simulink model "PlanarArmAug"  (R2025b)
settings: Solver=VariableStepAuto  StartTime=0.0  StopTime=10.0  RelTol=1e-3
undefined symbols (not defined in the file): InvDynAug, Jr, sig4, ureal, uss
libraries: RCTblocks x149
(part 1 of 2)
settings Model: Creator=d.alazard  LastModifiedBy=andre
settings SolverCC: AlgebraicLoopSolver=TrustRegion
settings DebuggingCC: AlgebraicLoopMsg=none  UnconnectedInputMsg=warning  UnconnectedOutputMsg=warning  UnconnectedLineMsg=warning
settings ModelReferenceCC: EnableRefExpFcnMdlSchedulingChecks=on
settings RTWCC: GPUComputeCapability=3.5  DLArmComputeVersion=19.05

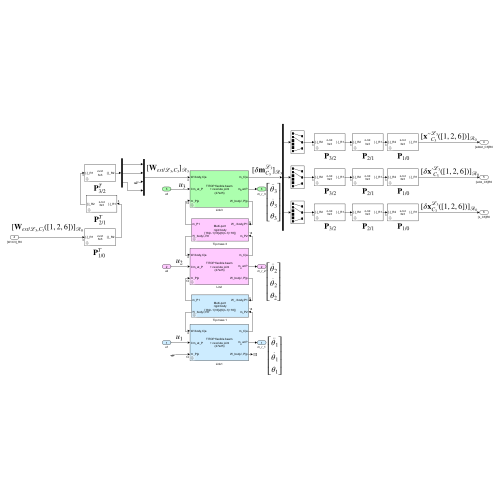
[thumbnail: Simulink's stored preview of the top-level diagram]
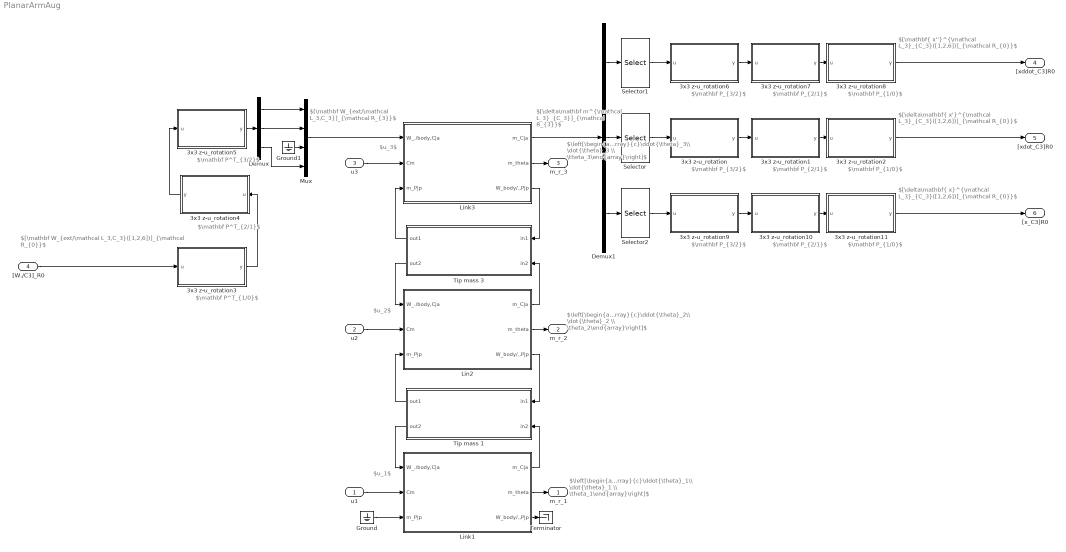
== system PlanarArmAug ==
  note: $[\delta\mathbf m^{\mathcal L_3}_{C_3}]_{\mathcal R_{3}}$
  note: $[\delta\mathbf{ x'}^{\mathcal L_3}_{C_3}([1,2,6])]_{\mathcal R_{0}}$
  note: $[\mathbf W_{ext/\mathcal L_3,C_3}]_{\mathcal R_{3}}$
  note: $[\mathbf W_{ext/\mathcal L_3,C_3}([1,2,6])]_{\mathcal R_{0}}$
  note: $u_3$
  note: $u_2$
  note: $u_1$
  note: $\left[\begin{array}{c}\ddot{\theta}_1\\ \dot{\theta}_1 \\ \theta_1\end{array}\right]$
  note: $\mathbf P_{3/2}$
  note: $\mathbf P^T_{2/1}$
  note: $\mathbf P_{1/0}$
  note: $\mathbf P^T_{1/0}$
  note: $\mathbf P_{2/1}$
  note: $\mathbf P^T_{3/2}$
  note: $\left[\begin{array}{c}\ddot{\theta}_2\\ \dot{\theta}_2 \\ \theta_2\end{array}\right]$
  note: $\left[\begin{array}{c}\ddot{\theta}_3\\ \dot{\theta}_3 \\ \theta_3\end{array}\right]$
  note: $[\mathbf{ x''}^{\mathcal L_3}_{C_3}([1,2,6])]_{\mathcal R_{0}}$
  note: $\mathbf P_{3/2}$
  note: $\mathbf P_{1/0}$
  note: $\mathbf P_{2/1}$
  note: $[\delta\mathbf{ x}^{\mathcal L_3}_{C_3}([1,2,6])]_{\mathcal R_{0}}$
  note: $\mathbf P_{3/2}$
  note: $\mathbf P_{1/0}$
  note: $\mathbf P_{2/1}$
  u1 : Inport
  u2 : Inport  Port=2
  u3 : Inport  Port=3
  "[W./C3]_R0" : Inport  Port=4
  3x3 z-u_rotation : Subsystem  mask(3x3 rotation matrix (around 3-rd axis)){theta=ureal('theta3',0,'Range',[-pi pi]), transp=off}
      mask prompts: theta "Angle (rad)"; transp "DCM transposed"
      mask help:
      | Implement the 3x3 direction cosine matrix or its transposed
      | (DCM=[cos(x)   -sin(x) 0;sin(x)  cos(x) 0;0 0 1])
      | associated to the rotation of a given angle x around the 3-rd axis.
      |
      | Angle  (rad) can be an uncertain parameter declared with "ureal" with mode 'Range'
      | Ex: ureal('NAME',0,'Range',[-pi pi])
      | Then, ULINEARIZE will provide a model involving the block named "tan_NAME_div4".
      mask init:
      | zUrotation3x3
      mask Help: web('Doc3zurotation.html','-browser')
      mask Display:
      | disp('z-rot\n3x3')
      | if transp
      |     port_label('input', 1, '[.]_R1')
      |     port_label('output', 1, '[.]_R2')
      | else
      |     port_label('input', 1, '[.]_R2')
      |     port_label('output', 1, '[.]_R1')
      | end
  3x3 z-u_rotation1 : Subsystem  mask(3x3 rotation matrix (around 3-rd axis)){theta=ureal('theta2',0,'Range',[-pi pi]), transp=off}
      mask prompts: theta "Angle (rad)"; transp "DCM transposed"
      mask help:
      | Implement the 3x3 direction cosine matrix or its transposed
      | (DCM=[cos(x)   -sin(x) 0;sin(x)  cos(x) 0;0 0 1])
      | associated to the rotation of a given angle x around the 3-rd axis.
      |
      | Angle  (rad) can be an uncertain parameter declared with "ureal" with mode 'Range'
      | Ex: ureal('NAME',0,'Range',[-pi pi])
      | Then, ULINEARIZE will provide a model involving the block named "tan_NAME_div4".
      mask init:
      | zUrotation3x3
      mask Help: web('Doc3zurotation.html','-browser')
      mask Display:
      | disp('z-rot\n3x3')
      | if transp
      |     port_label('input', 1, '[.]_R1')
      |     port_label('output', 1, '[.]_R2')
      | else
      |     port_label('input', 1, '[.]_R2')
      |     port_label('output', 1, '[.]_R1')
      | end
  3x3 z-u_rotation10 : Subsystem  mask(3x3 rotation matrix (around 3-rd axis)){theta=ureal('theta2',0,'Range',[-pi pi]), transp=off}
      mask prompts: theta "Angle (rad)"; transp "DCM transposed"
      mask help:
      | Implement the 3x3 direction cosine matrix or its transposed
      | (DCM=[cos(x)   -sin(x) 0;sin(x)  cos(x) 0;0 0 1])
      | associated to the rotation of a given angle x around the 3-rd axis.
      |
      | Angle  (rad) can be an uncertain parameter declared with "ureal" with mode 'Range'
      | Ex: ureal('NAME',0,'Range',[-pi pi])
      | Then, ULINEARIZE will provide a model involving the block named "tan_NAME_div4".
      mask init:
      | zUrotation3x3
      mask Help: web('Doc3zurotation.html','-browser')
      mask Display:
      | disp('z-rot\n3x3')
      | if transp
      |     port_label('input', 1, '[.]_R1')
      |     port_label('output', 1, '[.]_R2')
      | else
      |     port_label('input', 1, '[.]_R2')
      |     port_label('output', 1, '[.]_R1')
      | end
  3x3 z-u_rotation11 : Subsystem  mask(3x3 rotation matrix (around 3-rd axis)){theta=ureal('theta1',0,'Range',[-pi pi]), transp=off}
      mask prompts: theta "Angle (rad)"; transp "DCM transposed"
      mask help:
      | Implement the 3x3 direction cosine matrix or its transposed
      | (DCM=[cos(x)   -sin(x) 0;sin(x)  cos(x) 0;0 0 1])
      | associated to the rotation of a given angle x around the 3-rd axis.
      |
      | Angle  (rad) can be an uncertain parameter declared with "ureal" with mode 'Range'
      | Ex: ureal('NAME',0,'Range',[-pi pi])
      | Then, ULINEARIZE will provide a model involving the block named "tan_NAME_div4".
      mask init:
      | zUrotation3x3
      mask Help: web('Doc3zurotation.html','-browser')
      mask Display:
      | disp('z-rot\n3x3')
      | if transp
      |     port_label('input', 1, '[.]_R1')
      |     port_label('output', 1, '[.]_R2')
      | else
      |     port_label('input', 1, '[.]_R2')
      |     port_label('output', 1, '[.]_R1')
      | end
  3x3 z-u_rotation2 : Subsystem  mask(3x3 rotation matrix (around 3-rd axis)){theta=ureal('theta1',0,'Range',[-pi pi]), transp=off}
      mask prompts: theta "Angle (rad)"; transp "DCM transposed"
      mask help:
      | Implement the 3x3 direction cosine matrix or its transposed
      | (DCM=[cos(x)   -sin(x) 0;sin(x)  cos(x) 0;0 0 1])
      | associated to the rotation of a given angle x around the 3-rd axis.
      |
      | Angle  (rad) can be an uncertain parameter declared with "ureal" with mode 'Range'
      | Ex: ureal('NAME',0,'Range',[-pi pi])
      | Then, ULINEARIZE will provide a model involving the block named "tan_NAME_div4".
      mask init:
      | zUrotation3x3
      mask Help: web('Doc3zurotation.html','-browser')
      mask Display:
      | disp('z-rot\n3x3')
      | if transp
      |     port_label('input', 1, '[.]_R1')
      |     port_label('output', 1, '[.]_R2')
      | else
      |     port_label('input', 1, '[.]_R2')
      |     port_label('output', 1, '[.]_R1')
      | end
  3x3 z-u_rotation3 : Subsystem  mask(3x3 rotation matrix (around 3-rd axis)){theta=ureal('theta1',0,'Range',[-pi pi]), transp=on}
      mask prompts: theta "Angle (rad)"; transp "DCM transposed"
      mask help:
      | Implement the 3x3 direction cosine matrix or its transposed
      | (DCM=[cos(x)   -sin(x) 0;sin(x)  cos(x) 0;0 0 1])
      | associated to the rotation of a given angle x around the 3-rd axis.
      |
      | Angle  (rad) can be an uncertain parameter declared with "ureal" with mode 'Range'
      | Ex: ureal('NAME',0,'Range',[-pi pi])
      | Then, ULINEARIZE will provide a model involving the block named "tan_NAME_div4".
      mask init:
      | zUrotation3x3
      mask Help: web('Doc3zurotation.html','-browser')
      mask Display:
      | disp('z-rot\n3x3')
      | if transp
      |     port_label('input', 1, '[.]_R1')
      |     port_label('output', 1, '[.]_R2')
      | else
      |     port_label('input', 1, '[.]_R2')
      |     port_label('output', 1, '[.]_R1')
      | end
  3x3 z-u_rotation4 : Subsystem  mask(3x3 rotation matrix (around 3-rd axis)){theta=ureal('theta2',0,'Range',[-pi pi]), transp=on}
      mask prompts: theta "Angle (rad)"; transp "DCM transposed"
      mask help:
      | Implement the 3x3 direction cosine matrix or its transposed
      | (DCM=[cos(x)   -sin(x) 0;sin(x)  cos(x) 0;0 0 1])
      | associated to the rotation of a given angle x around the 3-rd axis.
      |
      | Angle  (rad) can be an uncertain parameter declared with "ureal" with mode 'Range'
      | Ex: ureal('NAME',0,'Range',[-pi pi])
      | Then, ULINEARIZE will provide a model involving the block named "tan_NAME_div4".
      mask init:
      | zUrotation3x3
      mask Help: web('Doc3zurotation.html','-browser')
      mask Display:
      | disp('z-rot\n3x3')
      | if transp
      |     port_label('input', 1, '[.]_R1')
      |     port_label('output', 1, '[.]_R2')
      | else
      |     port_label('input', 1, '[.]_R2')
      |     port_label('output', 1, '[.]_R1')
      | end
  3x3 z-u_rotation5 : Subsystem  mask(3x3 rotation matrix (around 3-rd axis)){theta=ureal('theta3',0,'Range',[-pi pi]), transp=on}
      mask prompts: theta "Angle (rad)"; transp "DCM transposed"
      mask help:
      | Implement the 3x3 direction cosine matrix or its transposed
      | (DCM=[cos(x)   -sin(x) 0;sin(x)  cos(x) 0;0 0 1])
      | associated to the rotation of a given angle x around the 3-rd axis.
      |
      | Angle  (rad) can be an uncertain parameter declared with "ureal" with mode 'Range'
      | Ex: ureal('NAME',0,'Range',[-pi pi])
      | Then, ULINEARIZE will provide a model involving the block named "tan_NAME_div4".
      mask init:
      | zUrotation3x3
      mask Help: web('Doc3zurotation.html','-browser')
      mask Display:
      | disp('z-rot\n3x3')
      | if transp
      |     port_label('input', 1, '[.]_R1')
      |     port_label('output', 1, '[.]_R2')
      | else
      |     port_label('input', 1, '[.]_R2')
      |     port_label('output', 1, '[.]_R1')
      | end
  3x3 z-u_rotation6 : Subsystem  mask(3x3 rotation matrix (around 3-rd axis)){theta=ureal('theta3',0,'Range',[-pi pi]), transp=off}
      mask prompts: theta "Angle (rad)"; transp "DCM transposed"
      mask help:
      | Implement the 3x3 direction cosine matrix or its transposed
      | (DCM=[cos(x)   -sin(x) 0;sin(x)  cos(x) 0;0 0 1])
      | associated to the rotation of a given angle x around the 3-rd axis.
      |
      | Angle  (rad) can be an uncertain parameter declared with "ureal" with mode 'Range'
      | Ex: ureal('NAME',0,'Range',[-pi pi])
      | Then, ULINEARIZE will provide a model involving the block named "tan_NAME_div4".
      mask init:
      | zUrotation3x3
      mask Help: web('Doc3zurotation.html','-browser')
      mask Display:
      | disp('z-rot\n3x3')
      | if transp
      |     port_label('input', 1, '[.]_R1')
      |     port_label('output', 1, '[.]_R2')
      | else
      |     port_label('input', 1, '[.]_R2')
      |     port_label('output', 1, '[.]_R1')
      | end
  3x3 z-u_rotation7 : Subsystem  mask(3x3 rotation matrix (around 3-rd axis)){theta=ureal('theta2',0,'Range',[-pi pi]), transp=off}
      mask prompts: theta "Angle (rad)"; transp "DCM transposed"
      mask help:
      | Implement the 3x3 direction cosine matrix or its transposed
      | (DCM=[cos(x)   -sin(x) 0;sin(x)  cos(x) 0;0 0 1])
      | associated to the rotation of a given angle x around the 3-rd axis.
      |
      | Angle  (rad) can be an uncertain parameter declared with "ureal" with mode 'Range'
      | Ex: ureal('NAME',0,'Range',[-pi pi])
      | Then, ULINEARIZE will provide a model involving the block named "tan_NAME_div4".
      mask init:
      | zUrotation3x3
      mask Help: web('Doc3zurotation.html','-browser')
      mask Display:
      | disp('z-rot\n3x3')
      | if transp
      |     port_label('input', 1, '[.]_R1')
      |     port_label('output', 1, '[.]_R2')
      | else
      |     port_label('input', 1, '[.]_R2')
      |     port_label('output', 1, '[.]_R1')
      | end
  3x3 z-u_rotation8 : Subsystem  mask(3x3 rotation matrix (around 3-rd axis)){theta=ureal('theta1',0,'Range',[-pi pi]), transp=off}
      mask prompts: theta "Angle (rad)"; transp "DCM transposed"
      mask help:
      | Implement the 3x3 direction cosine matrix or its transposed
      | (DCM=[cos(x)   -sin(x) 0;sin(x)  cos(x) 0;0 0 1])
      | associated to the rotation of a given angle x around the 3-rd axis.
      |
      | Angle  (rad) can be an uncertain parameter declared with "ureal" with mode 'Range'
      | Ex: ureal('NAME',0,'Range',[-pi pi])
      | Then, ULINEARIZE will provide a model involving the block named "tan_NAME_div4".
      mask init:
      | zUrotation3x3
      mask Help: web('Doc3zurotation.html','-browser')
      mask Display:
      | disp('z-rot\n3x3')
      | if transp
      |     port_label('input', 1, '[.]_R1')
      |     port_label('output', 1, '[.]_R2')
      | else
      |     port_label('input', 1, '[.]_R2')
      |     port_label('output', 1, '[.]_R1')
      | end
  3x3 z-u_rotation9 : Subsystem  mask(3x3 rotation matrix (around 3-rd axis)){theta=ureal('theta3',0,'Range',[-pi pi]), transp=off}
      mask prompts: theta "Angle (rad)"; transp "DCM transposed"
      mask help:
      | Implement the 3x3 direction cosine matrix or its transposed
      | (DCM=[cos(x)   -sin(x) 0;sin(x)  cos(x) 0;0 0 1])
      | associated to the rotation of a given angle x around the 3-rd axis.
      |
      | Angle  (rad) can be an uncertain parameter declared with "ureal" with mode 'Range'
      | Ex: ureal('NAME',0,'Range',[-pi pi])
      | Then, ULINEARIZE will provide a model involving the block named "tan_NAME_div4".
      mask init:
      | zUrotation3x3
      mask Help: web('Doc3zurotation.html','-browser')
      mask Display:
      | disp('z-rot\n3x3')
      | if transp
      |     port_label('input', 1, '[.]_R1')
      |     port_label('output', 1, '[.]_R2')
      | else
      |     port_label('input', 1, '[.]_R2')
      |     port_label('output', 1, '[.]_R1')
      | end
  Demux : Demux  Outputs=3
  Demux1 : Demux  Outputs=[6 6 6]
  Ground : Ground
  Ground1 : Ground
  Lin2 : Subsystem  mask(TITOP flexible beam with revolute joint (27x25)){l=1, s=0.01^2, rho=2700, E=69e9, Iz=0.01^4/12, Iy=0.01^4/12, ni=0.35, xi=0.001, Won=off, uw_var=10, Nflex=3, ra=[0;0;1], theta=ureal('theta2',0,'Range',[-pi pi])}
      mask prompts: l "length along x (m)"; s "cross section (m^2)"; rho "mass density (Kg/m^3)"; E "Young modulus (N/m^2)"; Iz "second moment of area along z axis, Iz (m^4)"; Iy "second moment of area along y axis Iy, (m^4)"; ni "Poisson coefficient"; xi "dampig ratio"; uw_var "uncertainty (d_w, %)"; Nflex "number of flexible mode (Nflex, integer<=10)"; ra "ra (joint axis) (3x1 vector)"; theta "angular configuration (rad)"
      mask help:
      | Computes the 27x25 model :
      | - 18x6 transfer from the wrenches applied to this body to the motion vector at port C,
      | - the 3x1 channel:
      |               * from  the  joint torque applied by the input (parent) shaft to the output (body) shaft
      |               * to the relative motion vector of the output shaft w.r.t the input shaft [thetaddot;thetadot;theta].
      | - 6x18 transfer from the motion vector to the wrench applied by this body to a parent body at port P through a revolute joint
      |
      | Input/Output of port P are expressed in the parent frame Rp
      | Input/Output of port C are expressed in the body frame Ra.
      |
      | ra: direction of the revolute joint in the Rp (or Ra)
      | theta: angular configuration of the joint (Ra is obtained from Rp by a rotation of theta around ra).
      |
      | All parameters must be expressed in the body frame Ra.
      | Each parameter can be an uncertain parameter declared with the function ureal (except ra)
      |
      | Rk: if "theta" field is: ureal('NAME',0,'Range',[-pi pi])
      | then, ULINEARIZE will provide a model involving the block named "tan_NAME_div4";
      mask init:
      | BeamRev2PortAug
      mask Help: web('DocBeamRevolute.html','-browser')
      mask DialogControl Container5 Prompt: Direct uncertainties on flexible mode frequencies
      mask DialogControl Control2 Prompt: Uncertainties on physical parameters (length, mass, ..) can create huge LFTs.
      mask DialogControl Control3 Prompt: Check this box to overwrite physical parameter uncertainties by a common relative uncertainty (d_w, %) on the first (Nflex) flexible mode frequencies of the clamped at P / free at C beam.
      mask DialogControl Control4 Prompt: The uncertain frequency is named: 'w_name_i' where:
      mask DialogControl Control5 Prompt: * 'name' is the current block name (reduced to its alphanumeric characters).
      mask DialogControl Control6 Prompt: * 'i' is the flexible mode number (increasing frequency order)
      mask DialogControl Container6 Prompt: Joint data
      mask Display:
      | disp('TITOP flexible beam\n + revolute joint\n (27x25)')
      | 
      | port_label('input', 1,'W./body,C|a')
      | port_label('output',1,'m_C|a')
      | port_label('input', 2,'Cm_at_P')
      | port_label('output',2,'m_\theta at P','interpreter','tex')
      | port_label('input', 3,'m_P|p')
      | port_label('output',3,'W_body/.,P|p')
  Link1 : Subsystem  mask(TITOP flexible beam with revolute joint (27x25)){l=1, s=0.01^2, rho=2700, E=69e9, Iz=0.01^4/12, Iy=0.01^4/12, ni=0.35, xi=0.001, Won=off, uw_var=10, Nflex=3, ra=[0;0;1], theta=ureal('theta1',0,'Range',[-pi pi])}
      mask prompts: l "length along x (m)"; s "cross section (m^2)"; rho "mass density (Kg/m^3)"; E "Young modulus (N/m^2)"; Iz "second moment of area along z axis, Iz (m^4)"; Iy "second moment of area along y axis Iy, (m^4)"; ni "Poisson coefficient"; xi "dampig ratio"; uw_var "uncertainty (d_w, %)"; Nflex "number of flexible mode (Nflex, integer<=10)"; ra "ra (joint axis) (3x1 vector)"; theta "angular configuration (rad)"
      mask help:
      | Computes the 27x25 model :
      | - 18x6 transfer from the wrenches applied to this body to the motion vector at port C,
      | - the 3x1 channel:
      |               * from  the  joint torque applied by the input (parent) shaft to the output (body) shaft
      |               * to the relative motion vector of the output shaft w.r.t the input shaft [thetaddot;thetadot;theta].
      | - 6x18 transfer from the motion vector to the wrench applied by this body to a parent body at port P through a revolute joint
      |
      | Input/Output of port P are expressed in the parent frame Rp
      | Input/Output of port C are expressed in the body frame Ra.
      |
      | ra: direction of the revolute joint in the Rp (or Ra)
      | theta: angular configuration of the joint (Ra is obtained from Rp by a rotation of theta around ra).
      |
      | All parameters must be expressed in the body frame Ra.
      | Each parameter can be an uncertain parameter declared with the function ureal (except ra)
      |
      | Rk: if "theta" field is: ureal('NAME',0,'Range',[-pi pi])
      | then, ULINEARIZE will provide a model involving the block named "tan_NAME_div4";
      mask init:
      | BeamRev2PortAug
      mask Help: web('DocBeamRevolute.html','-browser')
      mask DialogControl Container5 Prompt: Direct uncertainties on flexible mode frequencies
      mask DialogControl Control2 Prompt: Uncertainties on physical parameters (length, mass, ..) can create huge LFTs.
      mask DialogControl Control3 Prompt: Check this box to overwrite physical parameter uncertainties by a common relative uncertainty (d_w, %) on the first (Nflex) flexible mode frequencies of the clamped at P / free at C beam.
      mask DialogControl Control4 Prompt: The uncertain frequency is named: 'w_name_i' where:
      mask DialogControl Control5 Prompt: * 'name' is the current block name (reduced to its alphanumeric characters).
      mask DialogControl Control6 Prompt: * 'i' is the flexible mode number (increasing frequency order)
      mask DialogControl Container6 Prompt: Joint data
      mask Display:
      | disp('TITOP flexible beam\n + revolute joint\n (27x25)')
      | 
      | port_label('input', 1,'W./body,C|a')
      | port_label('output',1,'m_C|a')
      | port_label('input', 2,'Cm_at_P')
      | port_label('output',2,'m_\theta at P','interpreter','tex')
      | port_label('input', 3,'m_P|p')
      | port_label('output',3,'W_body/.,P|p')
  Link3 : Subsystem  mask(TITOP flexible beam with revolute joint (27x25)){l=1, s=0.01^2, rho=2700, E=69e9, Iz=0.01^4/12, Iy=0.01^4/12, ni=0.35, xi=0.001, Won=off, uw_var=10, Nflex=3, ra=[0;0;1], theta=ureal('theta3',0,'Range',[-pi pi])}
      mask prompts: l "length along x (m)"; s "cross section (m^2)"; rho "mass density (Kg/m^3)"; E "Young modulus (N/m^2)"; Iz "second moment of area along z axis, Iz (m^4)"; Iy "second moment of area along y axis Iy, (m^4)"; ni "Poisson coefficient"; xi "dampig ratio"; uw_var "uncertainty (d_w, %)"; Nflex "number of flexible mode (Nflex, integer<=10)"; ra "ra (joint axis) (3x1 vector)"; theta "angular configuration (rad)"
      mask help:
      | Computes the 27x25 model :
      | - 18x6 transfer from the wrenches applied to this body to the motion vector at port C,
      | - the 3x1 channel:
      |               * from  the  joint torque applied by the input (parent) shaft to the output (body) shaft
      |               * to the relative motion vector of the output shaft w.r.t the input shaft [thetaddot;thetadot;theta].
      | - 6x18 transfer from the motion vector to the wrench applied by this body to a parent body at port P through a revolute joint
      |
      | Input/Output of port P are expressed in the parent frame Rp
      | Input/Output of port C are expressed in the body frame Ra.
      |
      | ra: direction of the revolute joint in the Rp (or Ra)
      | theta: angular configuration of the joint (Ra is obtained from Rp by a rotation of theta around ra).
      |
      | All parameters must be expressed in the body frame Ra.
      | Each parameter can be an uncertain parameter declared with the function ureal (except ra)
      |
      | Rk: if "theta" field is: ureal('NAME',0,'Range',[-pi pi])
      | then, ULINEARIZE will provide a model involving the block named "tan_NAME_div4";
      mask init:
      | BeamRev2PortAug
      mask Help: web('DocBeamRevolute.html','-browser')
      mask DialogControl Container5 Prompt: Direct uncertainties on flexible mode frequencies
      mask DialogControl Control2 Prompt: Uncertainties on physical parameters (length, mass, ..) can create huge LFTs.
      mask DialogControl Control3 Prompt: Check this box to overwrite physical parameter uncertainties by a common relative uncertainty (d_w, %) on the first (Nflex) flexible mode frequencies of the clamped at P / free at C beam.
      mask DialogControl Control4 Prompt: The uncertain frequency is named: 'w_name_i' where:
      mask DialogControl Control5 Prompt: * 'name' is the current block name (reduced to its alphanumeric characters).
      mask DialogControl Control6 Prompt: * 'i' is the flexible mode number (increasing frequency order)
      mask DialogControl Container6 Prompt: Joint data
      mask Display:
      | disp('TITOP flexible beam\n + revolute joint\n (27x25)')
      | 
      | port_label('input', 1,'W./body,C|a')
      | port_label('output',1,'m_C|a')
      | port_label('input', 2,'Cm_at_P')
      | port_label('output',2,'m_\theta at P','interpreter','tex')
      | port_label('input', 3,'m_P|p')
      | port_label('output',3,'W_body/.,P|p')
  Mux : Mux  Inputs=[1 1 3 1]
  Selector : Selector  InputPortWidth=6  IndexOptions=Index vector (dialog)  Indices=[1 2 6]  OutputSizes=1
  Selector1 : Selector  InputPortWidth=6  IndexOptions=Index vector (dialog)  Indices=[1 2 6]  OutputSizes=1
  Selector2 : Selector  InputPortWidth=6  IndexOptions=Index vector (dialog)  Indices=[1 2 6]  OutputSizes=1
  Terminator : Terminator
  Tip mass 1 : Subsystem  mask(Multi-port rigid body (6nx6n)){m=1, Ig=zeros(3), OG=[0;0;0], n=2, numinv=2, OP1=[0;0;0], OP2=[0;0;0], OP3=[ureal('P3_y',1,'percent',10);0;0], OP4=[0;0;0], OP5=[0;0;0]}
      mask prompts: m "Mass (Kg)"; Ig "Inertia (at G, Kg m^2)"; OG "OG (3x1 vector, m)"; n "Number of ports"; numinv "Port to be inverted"; OP1 "OP1 (3x1 vector, m)"; OP2 "OP2 (3x1 vector, m)"; OP3 "OP3 (3x1 vector, m)"; OP4 "OP4 (3x1 vector, m)"; OP5 "OP5 (3x1 vector,m)"
      mask help:
      | 6nx6n dynamic model of a rigid body at n given points (ports) between wrenches applied at the n points (input) and acceleration twists at these points (output).
      |
      | 0: the reference point
      | G: the center of mass
      | Pi (i=1:n): the n given connection points (n<6).
      |
      | All parameters are expressed in the body frame.
      | Each parameter can be an uncertain parameter declared with "ureal"
      |
      | The 6x6 channel associated to one port can be inverted: then the input of this channel is the acceleration twist imposed at this point and the output is the wrench applied by this body.
      mask init:
      | MultiPortRigidBodyAug
      mask Help: web('Docmultiportrigidbody.html','-browser')
      mask TypeOptions n: 1 | 2 | 3 | 4 | 5
      mask TypeOptions numinv: 1 | 2 | 3 | 4 | 5
      mask DialogControl ParameterGroupVar Prompt: Main parameters
      mask DialogControl port1 Prompt: Port #1
      mask DialogControl port2 Prompt: #2
      mask DialogControl port3 Prompt: #3
      mask DialogControl port4 Prompt: #4
      mask DialogControl port5 Prompt: #5
      mask Display:
      | disp('Multi-port\n rigid body\n [18(n-1)+6]x[6(n-1)+18])')
      | if n==1,
      |     if numinv==1,
      |         port_label('input', 1,'m_P')
      |         port_label('output',1,'W_body/.,P')
      |     else
      |         port_label('input', 1,'W_./body,P')
      |         port_label('output',1,'m_P')
      |     end
      | else
      |     for ii=1:n
      |         if numinv==ii,
      |             port_label('output',ii,['W_body/.,P',num2str(ii)])
      |             port_label('input', ii,['m_P',num2str(ii)])
      |         else
      |             port_label('input', ii,['W_./body,P',num2str(ii)])
      |             port_label('output',ii,['m_P',num2str(ii)])
      |         end
      |     end
      | end
  Tip mass 3 : Subsystem  mask(Multi-port rigid body (6nx6n)){m=1, Ig=zeros(3), OG=[0;0;0], n=2, numinv=2, OP1=[0;0;0], OP2=[0;0;0], OP3=[ureal('P3_y',1,'percent',10);0;0], OP4=[0;0;0], OP5=[0;0;0]}
      mask prompts: m "Mass (Kg)"; Ig "Inertia (at G, Kg m^2)"; OG "OG (3x1 vector, m)"; n "Number of ports"; numinv "Port to be inverted"; OP1 "OP1 (3x1 vector, m)"; OP2 "OP2 (3x1 vector, m)"; OP3 "OP3 (3x1 vector, m)"; OP4 "OP4 (3x1 vector, m)"; OP5 "OP5 (3x1 vector,m)"
      mask help:
      | 6nx6n dynamic model of a rigid body at n given points (ports) between wrenches applied at the n points (input) and acceleration twists at these points (output).
      |
      | 0: the reference point
      | G: the center of mass
      | Pi (i=1:n): the n given connection points (n<6).
      |
      | All parameters are expressed in the body frame.
      | Each parameter can be an uncertain parameter declared with "ureal"
      |
      | The 6x6 channel associated to one port can be inverted: then the input of this channel is the acceleration twist imposed at this point and the output is the wrench applied by this body.
      mask init:
      | MultiPortRigidBodyAug
      mask Help: web('Docmultiportrigidbody.html','-browser')
      mask TypeOptions n: 1 | 2 | 3 | 4 | 5
      mask TypeOptions numinv: 1 | 2 | 3 | 4 | 5
      mask DialogControl ParameterGroupVar Prompt: Main parameters
      mask DialogControl port1 Prompt: Port #1
      mask DialogControl port2 Prompt: #2
      mask DialogControl port3 Prompt: #3
      mask DialogControl port4 Prompt: #4
      mask DialogControl port5 Prompt: #5
      mask Display:
      | disp('Multi-port\n rigid body\n [18(n-1)+6]x[6(n-1)+18])')
      | if n==1,
      |     if numinv==1,
      |         port_label('input', 1,'m_P')
      |         port_label('output',1,'W_body/.,P')
      |     else
      |         port_label('input', 1,'W_./body,P')
      |         port_label('output',1,'m_P')
      |     end
      | else
      |     for ii=1:n
      |         if numinv==ii,
      |             port_label('output',ii,['W_body/.,P',num2str(ii)])
      |             port_label('input', ii,['m_P',num2str(ii)])
      |         else
      |             port_label('input', ii,['W_./body,P',num2str(ii)])
      |             port_label('output',ii,['m_P',num2str(ii)])
      |         end
      |     end
      | end
  m_r_1 : Outport
  m_r_2 : Outport  Port=2
  m_r_3 : Outport  Port=3
  "[xddot_C3]R0" : Outport  Port=4
  "[xdot_C3]R0" : Outport  Port=5
  "[x_C3]R0" : Outport  Port=6
  wires:
  u1/1 -> Link1/2(Cm)
  Ground/1 -> Link1/3(m_P|p)
  Link1/3(W_body/.,P|p) -> Terminator/1
  Tip mass 1/2(out2) -> Link1/1(W_./body,C|a)
  Link1/1(m_C|a) -> Tip mass 1/2(in2)
  Tip mass 1/1(out1) -> Lin2/3(m_P|p)
  Lin2/3(W_body/.,P|p) -> Tip mass 1/1(in1)
  u2/1 -> Lin2/2(Cm)
  Lin2/1(m_C|a) -> Tip mass 3/2(in2)
  Tip mass 3/2(out2) -> Lin2/1(W_./body,C|a)
  u3/1 -> Link3/2(Cm)
  Tip mass 3/1(out1) -> Link3/3(m_P|p)
  Link3/3(W_body/.,P|p) -> Tip mass 3/1(in1)
  Ground1/1 -> Mux/3
  Demux/2 -> Mux/2
  Demux/3 -> Mux/4
  Mux/1 -> Link3/1(W_./body,C|a)
  Demux/1 -> Mux/1
  3x3 z-u_rotation2/1(y) -> "[xdot_C3]R0"/1
  Selector/1 -> 3x3 z-u_rotation/1(u)
  3x3 z-u_rotation3/1(y) -> 3x3 z-u_rotation4/1(u)
  "[W./C3]_R0"/1 -> 3x3 z-u_rotation3/1(u)
  3x3 z-u_rotation5/1(y) -> Demux/1
  3x3 z-u_rotation4/1(y) -> 3x3 z-u_rotation5/1(u)
  Link3/1(m_C|a) -> Demux1/1
  Lin2/2(m_theta) -> m_r_2/1
  Link1/2(m_theta) -> m_r_1/1
  Demux1/1 -> Selector1/1
  Demux1/2 -> Selector/1
  Link3/2(m_theta) -> m_r_3/1
  Demux1/3 -> Selector2/1
  3x3 z-u_rotation/1(y) -> 3x3 z-u_rotation1/1(u)
  3x3 z-u_rotation1/1(y) -> 3x3 z-u_rotation2/1(u)
  3x3 z-u_rotation7/1(y) -> 3x3 z-u_rotation8/1(u)
  3x3 z-u_rotation6/1(y) -> 3x3 z-u_rotation7/1(u)
  3x3 z-u_rotation8/1(y) -> "[xddot_C3]R0"/1
  Selector1/1 -> 3x3 z-u_rotation6/1(u)
  3x3 z-u_rotation10/1(y) -> 3x3 z-u_rotation11/1(u)
  3x3 z-u_rotation9/1(y) -> 3x3 z-u_rotation10/1(u)
  3x3 z-u_rotation11/1(y) -> "[x_C3]R0"/1
  Selector2/1 -> 3x3 z-u_rotation9/1(u)

== system PlanarArmAug/3x3 z-u_rotation ==
  u : Inport  PortDimensions=3
  Demux : Demux  Outputs=3
  Gain : Gain  Gain=2
  Gain1 : Gain  Gain=-2
  Gain2 : Gain  Gain=2
  Gain3 : Gain  Gain=2
  Mux : Mux  Inputs=3
  Sum : Sum  Inputs=++|
  Sum1 : Sum  Inputs=|++
  Sum2 : Sum  Inputs=|+-
  Sum3 : Sum  Inputs=|++
  Sum4 : Sum  Inputs=++|
  Sum5 : Sum  Inputs=++|
  Uncertain State Space{,1..3} (4 alike) : RCTblocks/Uncertain State Space  Tag=USS  USystem=uss(sig4)  UValue=[]  X0=[]  uX0=[]
  y : Outport  VectorParamsAs1DForOutWhenUnconnected=off
  wires:
  Demux/3 -> Mux/3
  Sum5/1 -> Gain2/1
  Uncertain State Space2/1 -> Uncertain State Space3/1, Sum2/2, Sum4/2
  Sum/1 -> Uncertain State Space/1
  Sum3/1 -> Uncertain State Space2/1
  Uncertain State Space/1 -> Uncertain State Space1/1, Sum5/1, Sum1/1
  Uncertain State Space1/1 -> Sum/1
  Gain3/1 -> Sum5/2
  Gain2/1 -> Sum3/1
  Demux/1 -> Gain3/1, Sum1/2
  Mux/1 -> y/1
  Uncertain State Space3/1 -> Sum3/2
  u/1 -> Demux/1
  Sum1/1 -> Mux/1
  Gain/1 -> Sum/2
  Demux/2 -> Gain1/1, Sum4/1
  Sum4/1 -> Mux/2
  Gain1/1 -> Sum2/1
  Sum2/1 -> Gain/1

== system PlanarArmAug/3x3 z-u_rotation1 ==
  u : Inport  PortDimensions=3
  Demux : Demux  Outputs=3
  Gain : Gain  Gain=2
  Gain1 : Gain  Gain=-2
  Gain2 : Gain  Gain=2
  Gain3 : Gain  Gain=2
  Mux : Mux  Inputs=3
  Sum : Sum  Inputs=++|
  Sum1 : Sum  Inputs=|++
  Sum2 : Sum  Inputs=|+-
  Sum3 : Sum  Inputs=|++
  Sum4 : Sum  Inputs=++|
  Sum5 : Sum  Inputs=++|
  Uncertain State Space{,1..3} (4 alike) : RCTblocks/Uncertain State Space  Tag=USS  USystem=uss(sig4)  UValue=[]  X0=[]  uX0=[]
  y : Outport  VectorParamsAs1DForOutWhenUnconnected=off
  wires:
  Demux/3 -> Mux/3
  Sum5/1 -> Gain2/1
  Uncertain State Space2/1 -> Uncertain State Space3/1, Sum2/2, Sum4/2
  Sum/1 -> Uncertain State Space/1
  Sum3/1 -> Uncertain State Space2/1
  Uncertain State Space/1 -> Uncertain State Space1/1, Sum5/1, Sum1/1
  Uncertain State Space1/1 -> Sum/1
  Gain3/1 -> Sum5/2
  Gain2/1 -> Sum3/1
  Demux/1 -> Gain3/1, Sum1/2
  Mux/1 -> y/1
  Uncertain State Space3/1 -> Sum3/2
  u/1 -> Demux/1
  Sum1/1 -> Mux/1
  Gain/1 -> Sum/2
  Demux/2 -> Gain1/1, Sum4/1
  Sum4/1 -> Mux/2
  Gain1/1 -> Sum2/1
  Sum2/1 -> Gain/1

== system PlanarArmAug/3x3 z-u_rotation10 ==
  u : Inport  PortDimensions=3
  Demux : Demux  Outputs=3
  Gain : Gain  Gain=2
  Gain1 : Gain  Gain=-2
  Gain2 : Gain  Gain=2
  Gain3 : Gain  Gain=2
  Mux : Mux  Inputs=3
  Sum : Sum  Inputs=++|
  Sum1 : Sum  Inputs=|++
  Sum2 : Sum  Inputs=|+-
  Sum3 : Sum  Inputs=|++
  Sum4 : Sum  Inputs=++|
  Sum5 : Sum  Inputs=++|
  Uncertain State Space{,1..3} (4 alike) : RCTblocks/Uncertain State Space  Tag=USS  USystem=uss(sig4)  UValue=[]  X0=[]  uX0=[]
  y : Outport  VectorParamsAs1DForOutWhenUnconnected=off
  wires:
  Sum2/1 -> Gain/1
  Gain1/1 -> Sum2/1
  Sum4/1 -> Mux/2
  Demux/2 -> Sum4/1, Gain1/1
  Gain/1 -> Sum/2
  Sum1/1 -> Mux/1
  u/1 -> Demux/1
  Uncertain State Space3/1 -> Sum3/2
  Mux/1 -> y/1
  Demux/1 -> Sum1/2, Gain3/1
  Gain2/1 -> Sum3/1
  Gain3/1 -> Sum5/2
  Uncertain State Space1/1 -> Sum/1
  Uncertain State Space/1 -> Sum1/1, Sum5/1, Uncertain State Space1/1
  Sum3/1 -> Uncertain State Space2/1
  Sum/1 -> Uncertain State Space/1
  Uncertain State Space2/1 -> Sum4/2, Sum2/2, Uncertain State Space3/1
  Sum5/1 -> Gain2/1
  Demux/3 -> Mux/3

== system PlanarArmAug/3x3 z-u_rotation11 ==
  u : Inport  PortDimensions=3
  Demux : Demux  Outputs=3
  Gain : Gain  Gain=2
  Gain1 : Gain  Gain=-2
  Gain2 : Gain  Gain=2
  Gain3 : Gain  Gain=2
  Mux : Mux  Inputs=3
  Sum : Sum  Inputs=++|
  Sum1 : Sum  Inputs=|++
  Sum2 : Sum  Inputs=|+-
  Sum3 : Sum  Inputs=|++
  Sum4 : Sum  Inputs=++|
  Sum5 : Sum  Inputs=++|
  Uncertain State Space{,1..3} (4 alike) : RCTblocks/Uncertain State Space  Tag=USS  USystem=uss(sig4)  UValue=[]  X0=[]  uX0=[]
  y : Outport  VectorParamsAs1DForOutWhenUnconnected=off
  wires:
  Sum2/1 -> Gain/1
  Gain1/1 -> Sum2/1
  Sum4/1 -> Mux/2
  Demux/2 -> Sum4/1, Gain1/1
  Gain/1 -> Sum/2
  Sum1/1 -> Mux/1
  u/1 -> Demux/1
  Uncertain State Space3/1 -> Sum3/2
  Mux/1 -> y/1
  Demux/1 -> Sum1/2, Gain3/1
  Gain2/1 -> Sum3/1
  Gain3/1 -> Sum5/2
  Uncertain State Space1/1 -> Sum/1
  Uncertain State Space/1 -> Sum1/1, Sum5/1, Uncertain State Space1/1
  Sum3/1 -> Uncertain State Space2/1
  Sum/1 -> Uncertain State Space/1
  Uncertain State Space2/1 -> Sum4/2, Sum2/2, Uncertain State Space3/1
  Sum5/1 -> Gain2/1
  Demux/3 -> Mux/3

== system PlanarArmAug/3x3 z-u_rotation2 ==
  u : Inport  PortDimensions=3
  Demux : Demux  Outputs=3
  Gain : Gain  Gain=2
  Gain1 : Gain  Gain=-2
  Gain2 : Gain  Gain=2
  Gain3 : Gain  Gain=2
  Mux : Mux  Inputs=3
  Sum : Sum  Inputs=++|
  Sum1 : Sum  Inputs=|++
  Sum2 : Sum  Inputs=|+-
  Sum3 : Sum  Inputs=|++
  Sum4 : Sum  Inputs=++|
  Sum5 : Sum  Inputs=++|
  Uncertain State Space{,1..3} (4 alike) : RCTblocks/Uncertain State Space  Tag=USS  USystem=uss(sig4)  UValue=[]  X0=[]  uX0=[]
  y : Outport  VectorParamsAs1DForOutWhenUnconnected=off
  wires:
  Demux/3 -> Mux/3
  Sum5/1 -> Gain2/1
  Uncertain State Space2/1 -> Uncertain State Space3/1, Sum2/2, Sum4/2
  Sum/1 -> Uncertain State Space/1
  Sum3/1 -> Uncertain State Space2/1
  Uncertain State Space/1 -> Uncertain State Space1/1, Sum5/1, Sum1/1
  Uncertain State Space1/1 -> Sum/1
  Gain3/1 -> Sum5/2
  Gain2/1 -> Sum3/1
  Demux/1 -> Gain3/1, Sum1/2
  Mux/1 -> y/1
  Uncertain State Space3/1 -> Sum3/2
  u/1 -> Demux/1
  Sum1/1 -> Mux/1
  Gain/1 -> Sum/2
  Demux/2 -> Gain1/1, Sum4/1
  Sum4/1 -> Mux/2
  Gain1/1 -> Sum2/1
  Sum2/1 -> Gain/1

== system PlanarArmAug/3x3 z-u_rotation3 ==
  u : Inport  PortDimensions=3
  Demux : Demux  Outputs=3
  Gain : Gain  Gain=2
  Gain1 : Gain  Gain=-2
  Gain2 : Gain  Gain=2
  Gain3 : Gain  Gain=2
  Mux : Mux  Inputs=3
  Sum : Sum  Inputs=++|
  Sum1 : Sum  Inputs=|++
  Sum2 : Sum  Inputs=|+-
  Sum3 : Sum  Inputs=|++
  Sum4 : Sum  Inputs=++|
  Sum5 : Sum  Inputs=++|
  Uncertain State Space{,1..3} (4 alike) : RCTblocks/Uncertain State Space  Tag=USS  USystem=uss(sig4)  UValue=[]  X0=[]  uX0=[]
  y : Outport  VectorParamsAs1DForOutWhenUnconnected=off
  wires:
  Demux/3 -> Mux/3
  Sum5/1 -> Gain2/1
  Uncertain State Space2/1 -> Uncertain State Space3/1, Sum2/2, Sum4/2
  Sum/1 -> Uncertain State Space/1
  Sum3/1 -> Uncertain State Space2/1
  Uncertain State Space/1 -> Uncertain State Space1/1, Sum5/1, Sum1/1
  Uncertain State Space1/1 -> Sum/1
  Gain3/1 -> Sum5/2
  Gain2/1 -> Sum3/1
  Demux/1 -> Gain3/1, Sum1/2
  Mux/1 -> y/1
  Uncertain State Space3/1 -> Sum3/2
  u/1 -> Demux/1
  Sum1/1 -> Mux/1
  Gain/1 -> Sum/2
  Demux/2 -> Gain1/1, Sum4/1
  Sum4/1 -> Mux/2
  Gain1/1 -> Sum2/1
  Sum2/1 -> Gain/1

== system PlanarArmAug/3x3 z-u_rotation4 ==
  u : Inport  PortDimensions=3
  Demux : Demux  Outputs=3
  Gain : Gain  Gain=2
  Gain1 : Gain  Gain=-2
  Gain2 : Gain  Gain=2
  Gain3 : Gain  Gain=2
  Mux : Mux  Inputs=3
  Sum : Sum  Inputs=++|
  Sum1 : Sum  Inputs=|++
  Sum2 : Sum  Inputs=|+-
  Sum3 : Sum  Inputs=|++
  Sum4 : Sum  Inputs=++|
  Sum5 : Sum  Inputs=++|
  Uncertain State Space{,1..3} (4 alike) : RCTblocks/Uncertain State Space  Tag=USS  USystem=uss(sig4)  UValue=[]  X0=[]  uX0=[]
  y : Outport  VectorParamsAs1DForOutWhenUnconnected=off
  wires:
  Demux/3 -> Mux/3
  Sum5/1 -> Gain2/1
  Uncertain State Space2/1 -> Uncertain State Space3/1, Sum2/2, Sum4/2
  Sum/1 -> Uncertain State Space/1
  Sum3/1 -> Uncertain State Space2/1
  Uncertain State Space/1 -> Uncertain State Space1/1, Sum5/1, Sum1/1
  Uncertain State Space1/1 -> Sum/1
  Gain3/1 -> Sum5/2
  Gain2/1 -> Sum3/1
  Demux/1 -> Gain3/1, Sum1/2
  Mux/1 -> y/1
  Uncertain State Space3/1 -> Sum3/2
  u/1 -> Demux/1
  Sum1/1 -> Mux/1
  Gain/1 -> Sum/2
  Demux/2 -> Gain1/1, Sum4/1
  Sum4/1 -> Mux/2
  Gain1/1 -> Sum2/1
  Sum2/1 -> Gain/1

== system PlanarArmAug/3x3 z-u_rotation5 ==
  u : Inport  PortDimensions=3
  Demux : Demux  Outputs=3
  Gain : Gain  Gain=2
  Gain1 : Gain  Gain=-2
  Gain2 : Gain  Gain=2
  Gain3 : Gain  Gain=2
  Mux : Mux  Inputs=3
  Sum : Sum  Inputs=++|
  Sum1 : Sum  Inputs=|++
  Sum2 : Sum  Inputs=|+-
  Sum3 : Sum  Inputs=|++
  Sum4 : Sum  Inputs=++|
  Sum5 : Sum  Inputs=++|
  Uncertain State Space{,1..3} (4 alike) : RCTblocks/Uncertain State Space  Tag=USS  USystem=uss(sig4)  UValue=[]  X0=[]  uX0=[]
  y : Outport  VectorParamsAs1DForOutWhenUnconnected=off
  wires:
  Demux/3 -> Mux/3
  Sum5/1 -> Gain2/1
  Uncertain State Space2/1 -> Uncertain State Space3/1, Sum2/2, Sum4/2
  Sum/1 -> Uncertain State Space/1
  Sum3/1 -> Uncertain State Space2/1
  Uncertain State Space/1 -> Uncertain State Space1/1, Sum5/1, Sum1/1
  Uncertain State Space1/1 -> Sum/1
  Gain3/1 -> Sum5/2
  Gain2/1 -> Sum3/1
  Demux/1 -> Gain3/1, Sum1/2
  Mux/1 -> y/1
  Uncertain State Space3/1 -> Sum3/2
  u/1 -> Demux/1
  Sum1/1 -> Mux/1
  Gain/1 -> Sum/2
  Demux/2 -> Gain1/1, Sum4/1
  Sum4/1 -> Mux/2
  Gain1/1 -> Sum2/1
  Sum2/1 -> Gain/1

== system PlanarArmAug/3x3 z-u_rotation6 ==
  u : Inport  PortDimensions=3
  Demux : Demux  Outputs=3
  Gain : Gain  Gain=2
  Gain1 : Gain  Gain=-2
  Gain2 : Gain  Gain=2
  Gain3 : Gain  Gain=2
  Mux : Mux  Inputs=3
  Sum : Sum  Inputs=++|
  Sum1 : Sum  Inputs=|++
  Sum2 : Sum  Inputs=|+-
  Sum3 : Sum  Inputs=|++
  Sum4 : Sum  Inputs=++|
  Sum5 : Sum  Inputs=++|
  Uncertain State Space{,1..3} (4 alike) : RCTblocks/Uncertain State Space  Tag=USS  USystem=uss(sig4)  UValue=[]  X0=[]  uX0=[]
  y : Outport  VectorParamsAs1DForOutWhenUnconnected=off
  wires:
  Sum2/1 -> Gain/1
  Gain1/1 -> Sum2/1
  Sum4/1 -> Mux/2
  Demux/2 -> Sum4/1, Gain1/1
  Gain/1 -> Sum/2
  Sum1/1 -> Mux/1
  u/1 -> Demux/1
  Uncertain State Space3/1 -> Sum3/2
  Mux/1 -> y/1
  Demux/1 -> Sum1/2, Gain3/1
  Gain2/1 -> Sum3/1
  Gain3/1 -> Sum5/2
  Uncertain State Space1/1 -> Sum/1
  Uncertain State Space/1 -> Sum1/1, Sum5/1, Uncertain State Space1/1
  Sum3/1 -> Uncertain State Space2/1
  Sum/1 -> Uncertain State Space/1
  Uncertain State Space2/1 -> Sum4/2, Sum2/2, Uncertain State Space3/1
  Sum5/1 -> Gain2/1
  Demux/3 -> Mux/3

== system PlanarArmAug/3x3 z-u_rotation7 ==
  u : Inport  PortDimensions=3
  Demux : Demux  Outputs=3
  Gain : Gain  Gain=2
  Gain1 : Gain  Gain=-2
  Gain2 : Gain  Gain=2
  Gain3 : Gain  Gain=2
  Mux : Mux  Inputs=3
  Sum : Sum  Inputs=++|
  Sum1 : Sum  Inputs=|++
  Sum2 : Sum  Inputs=|+-
  Sum3 : Sum  Inputs=|++
  Sum4 : Sum  Inputs=++|
  Sum5 : Sum  Inputs=++|
  Uncertain State Space{,1..3} (4 alike) : RCTblocks/Uncertain State Space  Tag=USS  USystem=uss(sig4)  UValue=[]  X0=[]  uX0=[]
  y : Outport  VectorParamsAs1DForOutWhenUnconnected=off
  wires:
  Sum2/1 -> Gain/1
  Gain1/1 -> Sum2/1
  Sum4/1 -> Mux/2
  Demux/2 -> Sum4/1, Gain1/1
  Gain/1 -> Sum/2
  Sum1/1 -> Mux/1
  u/1 -> Demux/1
  Uncertain State Space3/1 -> Sum3/2
  Mux/1 -> y/1
  Demux/1 -> Sum1/2, Gain3/1
  Gain2/1 -> Sum3/1
  Gain3/1 -> Sum5/2
  Uncertain State Space1/1 -> Sum/1
  Uncertain State Space/1 -> Sum1/1, Sum5/1, Uncertain State Space1/1
  Sum3/1 -> Uncertain State Space2/1
  Sum/1 -> Uncertain State Space/1
  Uncertain State Space2/1 -> Sum4/2, Sum2/2, Uncertain State Space3/1
  Sum5/1 -> Gain2/1
  Demux/3 -> Mux/3

== system PlanarArmAug/3x3 z-u_rotation8 ==
  u : Inport  PortDimensions=3
  Demux : Demux  Outputs=3
  Gain : Gain  Gain=2
  Gain1 : Gain  Gain=-2
  Gain2 : Gain  Gain=2
  Gain3 : Gain  Gain=2
  Mux : Mux  Inputs=3
  Sum : Sum  Inputs=++|
  Sum1 : Sum  Inputs=|++
  Sum2 : Sum  Inputs=|+-
  Sum3 : Sum  Inputs=|++
  Sum4 : Sum  Inputs=++|
  Sum5 : Sum  Inputs=++|
  Uncertain State Space{,1..3} (4 alike) : RCTblocks/Uncertain State Space  Tag=USS  USystem=uss(sig4)  UValue=[]  X0=[]  uX0=[]
  y : Outport  VectorParamsAs1DForOutWhenUnconnected=off
  wires:
  Sum2/1 -> Gain/1
  Gain1/1 -> Sum2/1
  Sum4/1 -> Mux/2
  Demux/2 -> Sum4/1, Gain1/1
  Gain/1 -> Sum/2
  Sum1/1 -> Mux/1
  u/1 -> Demux/1
  Uncertain State Space3/1 -> Sum3/2
  Mux/1 -> y/1
  Demux/1 -> Sum1/2, Gain3/1
  Gain2/1 -> Sum3/1
  Gain3/1 -> Sum5/2
  Uncertain State Space1/1 -> Sum/1
  Uncertain State Space/1 -> Sum1/1, Sum5/1, Uncertain State Space1/1
  Sum3/1 -> Uncertain State Space2/1
  Sum/1 -> Uncertain State Space/1
  Uncertain State Space2/1 -> Sum4/2, Sum2/2, Uncertain State Space3/1
  Sum5/1 -> Gain2/1
  Demux/3 -> Mux/3

== system PlanarArmAug/3x3 z-u_rotation9 ==
  u : Inport  PortDimensions=3
  Demux : Demux  Outputs=3
  Gain : Gain  Gain=2
  Gain1 : Gain  Gain=-2
  Gain2 : Gain  Gain=2
  Gain3 : Gain  Gain=2
  Mux : Mux  Inputs=3
  Sum : Sum  Inputs=++|
  Sum1 : Sum  Inputs=|++
  Sum2 : Sum  Inputs=|+-
  Sum3 : Sum  Inputs=|++
  Sum4 : Sum  Inputs=++|
  Sum5 : Sum  Inputs=++|
  Uncertain State Space{,1..3} (4 alike) : RCTblocks/Uncertain State Space  Tag=USS  USystem=uss(sig4)  UValue=[]  X0=[]  uX0=[]
  y : Outport  VectorParamsAs1DForOutWhenUnconnected=off
  wires:
  Sum2/1 -> Gain/1
  Gain1/1 -> Sum2/1
  Sum4/1 -> Mux/2
  Demux/2 -> Sum4/1, Gain1/1
  Gain/1 -> Sum/2
  Sum1/1 -> Mux/1
  u/1 -> Demux/1
  Uncertain State Space3/1 -> Sum3/2
  Mux/1 -> y/1
  Demux/1 -> Sum1/2, Gain3/1
  Gain2/1 -> Sum3/1
  Gain3/1 -> Sum5/2
  Uncertain State Space1/1 -> Sum/1
  Uncertain State Space/1 -> Sum1/1, Sum5/1, Uncertain State Space1/1
  Sum3/1 -> Uncertain State Space2/1
  Sum/1 -> Uncertain State Space/1
  Uncertain State Space2/1 -> Sum4/2, Sum2/2, Uncertain State Space3/1
  Sum5/1 -> Gain2/1
  Demux/3 -> Mux/3

== system PlanarArmAug/Lin2 ==
  W_./body,C|a : Inport  PortDimensions=6
  Cm : Inport  Port=2
  m_P|p : Inport  Port=3  PortDimensions=18
  Demux : Demux  Outputs=[18 6]
      settings: DisplayOption=none
  Mux : Mux  Inputs=[6 18]
  Revolute joint + configuration : Subsystem  mask(Revolute joint){ra=ra, Jr=Jr, theta=theta}
      mask prompts: ra "Direction of the joint in the local frame (3x1 vector)"; Jr "Rotor inertia (kg.m^2)"; theta "Angular configuration (rad)"
      mask help:
      | This block implement the TITOP model of of a revolute joint.
      | The last channel is the transfer between the torque applied inside the joint by the input shaft to the output shaft and the relative angular acceleration of the output shaft w.r.t the input shaft.
      |
      | Angular configuration can be a vayring parameter: Ex:
      | ureal('NAME',0,'Range',[-pi pi])
      |
      | Then, ULINEARIZE will provide a model involving the block named "tan_NAME_div4";
      mask init:
      | pass=ra2DCMi(ra);
      | ran=[ra(1);ra(2);ra(3)]/norm(ra);
      mask Help: web('DocRevoluteJoint_configuration.html','-browser')
      mask Display:
      | disp('Revolute joint\nTITOP model\n+ angle configuration')
      | port_label('input', 1, 'W_./r_out|a')
      | port_label('output', 1, 'm_out|a')
      | port_label('input', 2, 'm_in|p')
      | port_label('output', 2, 'W_r_in/.|p')
      | port_label('input', 3, 'Cm')
      | port_label('output', 3, 'm_\theta','interpreter','tex')
  Uncertain State Space : RCTblocks/Uncertain State Space  Tag=USS  USystem=TITOPBEAM  UValue=[]  X0=[]  uX0=[]
  m_C|a : Outport  VectorParamsAs1DForOutWhenUnconnected=off
  m_theta : Outport  Port=2  VectorParamsAs1DForOutWhenUnconnected=off
  W_body/.,P|p : Outport  Port=3  VectorParamsAs1DForOutWhenUnconnected=off
  wires:
  Cm/1 -> Revolute joint + configuration/3(Cm)
  Revolute joint + configuration/1(m_out|a) -> Mux/2
  Revolute joint + configuration/2(W_r_in/.|p) -> W_body/.,P|p/1
  Revolute joint + configuration/3(m_theta) -> m_theta/1
  m_P|p/1 -> Revolute joint + configuration/2(m_in|p)
  Demux/2 -> Revolute joint + configuration/1(W_./r_out|a)
  Demux/1 -> m_C|a/1
  W_./body,C|a/1 -> Mux/1
  Mux/1 -> Uncertain State Space/1
  Uncertain State Space/1 -> Demux/1

== system PlanarArmAug/Link1 ==
  W_./body,C|a : Inport  PortDimensions=6
  Cm : Inport  Port=2
  m_P|p : Inport  Port=3  PortDimensions=18
  Demux : Demux  Outputs=[18 6]
      settings: DisplayOption=none
  Mux : Mux  Inputs=[6 18]
  Revolute joint + configuration : Subsystem  mask(Revolute joint){ra=ra, Jr=Jr, theta=theta}
      mask prompts: ra "Direction of the joint in the local frame (3x1 vector)"; Jr "Rotor inertia (kg.m^2)"; theta "Angular configuration (rad)"
      mask help:
      | This block implement the TITOP model of of a revolute joint.
      | The last channel is the transfer between the torque applied inside the joint by the input shaft to the output shaft and the relative angular acceleration of the output shaft w.r.t the input shaft.
      |
      | Angular configuration can be a vayring parameter: Ex:
      | ureal('NAME',0,'Range',[-pi pi])
      |
      | Then, ULINEARIZE will provide a model involving the block named "tan_NAME_div4";
      mask init:
      | pass=ra2DCMi(ra);
      | ran=[ra(1);ra(2);ra(3)]/norm(ra);
      mask Help: web('DocRevoluteJoint_configuration.html','-browser')
      mask Display:
      | disp('Revolute joint\nTITOP model\n+ angle configuration')
      | port_label('input', 1, 'W_./r_out|a')
      | port_label('output', 1, 'm_out|a')
      | port_label('input', 2, 'm_in|p')
      | port_label('output', 2, 'W_r_in/.|p')
      | port_label('input', 3, 'Cm')
      | port_label('output', 3, 'm_\theta','interpreter','tex')
  Uncertain State Space : RCTblocks/Uncertain State Space  Tag=USS  USystem=TITOPBEAM  UValue=[]  X0=[]  uX0=[]
  m_C|a : Outport  VectorParamsAs1DForOutWhenUnconnected=off
  m_theta : Outport  Port=2  VectorParamsAs1DForOutWhenUnconnected=off
  W_body/.,P|p : Outport  Port=3  VectorParamsAs1DForOutWhenUnconnected=off
  wires:
  Uncertain State Space/1 -> Demux/1
  Mux/1 -> Uncertain State Space/1
  W_./body,C|a/1 -> Mux/1
  Demux/1 -> m_C|a/1
  Demux/2 -> Revolute joint + configuration/1(W_./r_out|a)
  m_P|p/1 -> Revolute joint + configuration/2(m_in|p)
  Revolute joint + configuration/3(m_theta) -> m_theta/1
  Revolute joint + configuration/2(W_r_in/.|p) -> W_body/.,P|p/1
  Revolute joint + configuration/1(m_out|a) -> Mux/2
  Cm/1 -> Revolute joint + configuration/3(Cm)

== system PlanarArmAug/Link3 ==
  W_./body,C|a : Inport  PortDimensions=6
  Cm : Inport  Port=2
  m_P|p : Inport  Port=3  PortDimensions=18
  Demux : Demux  Outputs=[18 6]
      settings: DisplayOption=none
  Mux : Mux  Inputs=[6 18]
  Revolute joint + configuration : Subsystem  mask(Revolute joint){ra=ra, Jr=Jr, theta=theta}
      mask prompts: ra "Direction of the joint in the local frame (3x1 vector)"; Jr "Rotor inertia (kg.m^2)"; theta "Angular configuration (rad)"
      mask help:
      | This block implement the TITOP model of of a revolute joint.
      | The last channel is the transfer between the torque applied inside the joint by the input shaft to the output shaft and the relative angular acceleration of the output shaft w.r.t the input shaft.
      |
      | Angular configuration can be a vayring parameter: Ex:
      | ureal('NAME',0,'Range',[-pi pi])
      |
      | Then, ULINEARIZE will provide a model involving the block named "tan_NAME_div4";
      mask init:
      | pass=ra2DCMi(ra);
      | ran=[ra(1);ra(2);ra(3)]/norm(ra);
      mask Help: web('DocRevoluteJoint_configuration.html','-browser')
      mask Display:
      | disp('Revolute joint\nTITOP model\n+ angle configuration')
      | port_label('input', 1, 'W_./r_out|a')
      | port_label('output', 1, 'm_out|a')
      | port_label('input', 2, 'm_in|p')
      | port_label('output', 2, 'W_r_in/.|p')
      | port_label('input', 3, 'Cm')
      | port_label('output', 3, 'm_\theta','interpreter','tex')
  Uncertain State Space : RCTblocks/Uncertain State Space  Tag=USS  USystem=TITOPBEAM  UValue=[]  X0=[]  uX0=[]
  m_C|a : Outport  VectorParamsAs1DForOutWhenUnconnected=off
  m_theta : Outport  Port=2  VectorParamsAs1DForOutWhenUnconnected=off
  W_body/.,P|p : Outport  Port=3  VectorParamsAs1DForOutWhenUnconnected=off
  wires:
  Cm/1 -> Revolute joint + configuration/3(Cm)
  Revolute joint + configuration/1(m_out|a) -> Mux/2
  Revolute joint + configuration/2(W_r_in/.|p) -> W_body/.,P|p/1
  Revolute joint + configuration/3(m_theta) -> m_theta/1
  m_P|p/1 -> Revolute joint + configuration/2(m_in|p)
  Demux/2 -> Revolute joint + configuration/1(W_./r_out|a)
  Demux/1 -> m_C|a/1
  W_./body,C|a/1 -> Mux/1
  Mux/1 -> Uncertain State Space/1
  Uncertain State Space/1 -> Demux/1

== system PlanarArmAug/Tip mass 1 ==
  in1 : Inport  PortDimensions=6
  in2 : Inport  Port=2  PortDimensions=18
  Demux : Demux  Outputs=[ 18 6]
  Gain : RCTblocks/Uncertain State Space  Tag=USS  USystem=uss(InvDynAug)  UValue=[]  X0=[]  uX0=[]
  Mux : Mux  Inputs=[ 6 18]
  out1 : Outport
  out2 : Outport  Port=2
  wires:
  Mux/1 -> Gain/1
  Gain/1 -> Demux/1
  in1/1 -> Mux/1
  Demux/1 -> out1/1
  in2/1 -> Mux/2
  Demux/2 -> out2/1

== system PlanarArmAug/Tip mass 3 ==
  in1 : Inport  PortDimensions=6
  in2 : Inport  Port=2  PortDimensions=18
  Demux : Demux  Outputs=[ 18 6]
  Gain : RCTblocks/Uncertain State Space  Tag=USS  USystem=uss(InvDynAug)  UValue=[]  X0=[]  uX0=[]
  Mux : Mux  Inputs=[ 6 18]
  out1 : Outport
  out2 : Outport  Port=2
  wires:
  Demux/2 -> out2/1
  in2/1 -> Mux/2
  Demux/1 -> out1/1
  in1/1 -> Mux/1
  Gain/1 -> Demux/1
  Mux/1 -> Gain/1
